simulink model "rete_anticipatrice_ritardatrice"  (R2021a)
settings: Solver=VariableStepAuto  StartTime=0.0  StopTime=10.0  RelTol=1e-3
libraries: cstblocks x3, simulink x1
settings Model: Creator=itama  LastModifiedBy=itama

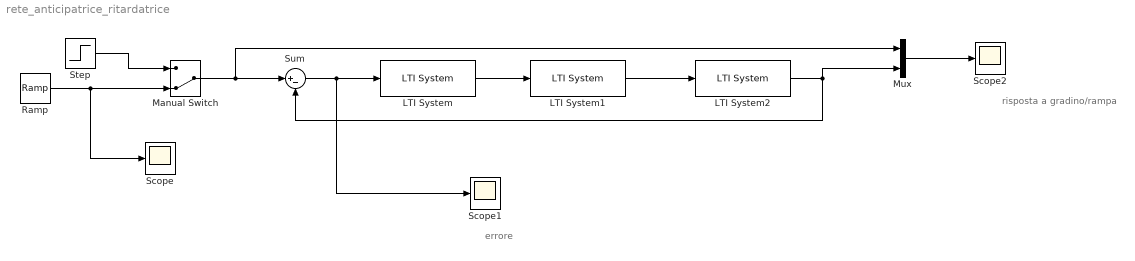
== system rete_anticipatrice_ritardatrice ==
  note: errore
  note: risposta a gradino/rampa
  LTI System : cstblocks/LTI System  sys=C1  IC=[]
  LTI System1 : cstblocks/LTI System  sys=C2  IC=[]
  LTI System2 : cstblocks/LTI System  sys=G  IC=[]
  Manual Switch : ManualSwitch  CurrentSetting=0
  Mux : Mux  Inputs=2
  Ramp : simulink/Sources/Ramp  slope=1  start=0  InitialOutput=0
  Scope : Scope
  Scope1 : Scope
  Scope2 : Scope
  Step : Step  Before=1  SampleTime=0
  Sum : Sum  Inputs=|+-
  wires:
  Step/1 -> Manual Switch/1
  Ramp/1 -> Scope/1, Manual Switch/2
  Manual Switch/1 -> Mux/1, Sum/1
  LTI System1/1 -> LTI System2/1
  Sum/1 -> Scope1/1, LTI System/1
  LTI System/1 -> LTI System1/1
  LTI System2/1 -> Sum/2, Mux/2
  Mux/1 -> Scope2/1
